simulink model "wetmodel"  (R2019b)
settings: Solver=ode45  StartTime=0.0  StopTime=10  RelTol=1e-3  EnableMultiTasking=on
model workspace (MAT data in the model file):
  SB_TRANSCOEFF = [1 10.1 101]
values from neighbouring files (symbols this model uses):
  B_thruster = [pi/2 0.05 0]    [Model_driver.m]
  Kd_x = 0    [Model_driver.m]
  Kd_y = 0    [Model_driver.m]
  Kd_yaw = 0    [Model_driver.m]
  Ki_x = 0    [Model_driver.m]
  Ki_y = 0    [Model_driver.m]
  Ki_yaw = 0    [Model_driver.m]
  Kp_x = 10    [Model_driver.m]
  Kp_y = 10    [Model_driver.m]
  Kp_yaw = 10    [Model_driver.m]
  P_thruster = [pi/2 -0.05 -0.05]    [Model_driver.m]
  SB_D = 10    [Model_driver.m]
  SB_I = 10    [Model_driver.m]
  SB_P = 10    [Model_driver.m]
  SB_thruster = [0 -0.05 0.05]    [Model_driver.m]
undefined symbols (not defined in the file or in its folder): IsPositionTracked, IsSkeletonTracked, JointDepthIndices, JointImageIndices, JointTrackingState, JointWorldCoordinates, magnitude, none, PositionDepthIndices, PositionImageIndices, PositionWorldCoordinates, Rec, SDTV, SegmentationData, SkeletonTrackingID, videoinput
libraries: powerlib_meascontrol x8, simulink x3, visionconversions x2, imaqlib x1, visionstatistics x1, visionsinks x1
settings Model: Tag=MP_system  Creator=Andries  LastModifiedBy=odend
settings DataIOCC: LimitDataPoints=on  SaveFormat=Array  SignalLoggingSaveFormat=ModelDataLogs  ReturnWorkspaceOutputs=off
settings OptimizationCC: ExpressionDepthLimit=2147483647  LifeSpan=inf
settings DebuggingCC: UnderspecifiedInitializationDetection=Classic  MergeDetectMultiDrivingBlocksExec=none  SolverPrmCheckMsg=warning  FcnCallInpInsideContextMsg=warning  StateNameClashWarn=warning  SFUnexpectedBacktrackingDiag=warning  SFNoUnconditionalDefaultTransitionDiag=warning  SFExecutionAtInitializationDiag=none  ArithmeticOperatorsInVariantConditions=warning
settings HardwareCC: ProdBitPerPointer=32  ProdBitPerSizeT=32  ProdBitPerPtrDiffT=32  ProdLargestAtomicFloat=None  ProdIntDivRoundTo=Undefined  ProdEndianess=Unspecified  ProdWordSize=32  ProdHWDeviceType=32-bit Generic
settings ModelReferenceCC: PropagateSignalLabelsOutOfModel=off
settings SFSimCC: SimUseLocalCustomCode=off  CustomCodeUndefinedFunction=UseInterfaceOnly
settings RTWCC: RTWUseLocalCustomCode=off
settings CodeAppCC: StateflowObjectComments=on
settings GRTTargetCC: TargetLangStandard=C89/C90 (ANSI)  GeneratePreprocessorConditionals=Disable all  CombineOutputUpdateFcns=off  GRTInterface=on
settings ConfigComp: CovMetricSettings=dw  CovHtmlReporting=on  CovSaveCumulativeToWorkspaceVar=on  CovSaveSingleToWorkspaceVar=on  CovExternalEMLEnable=off

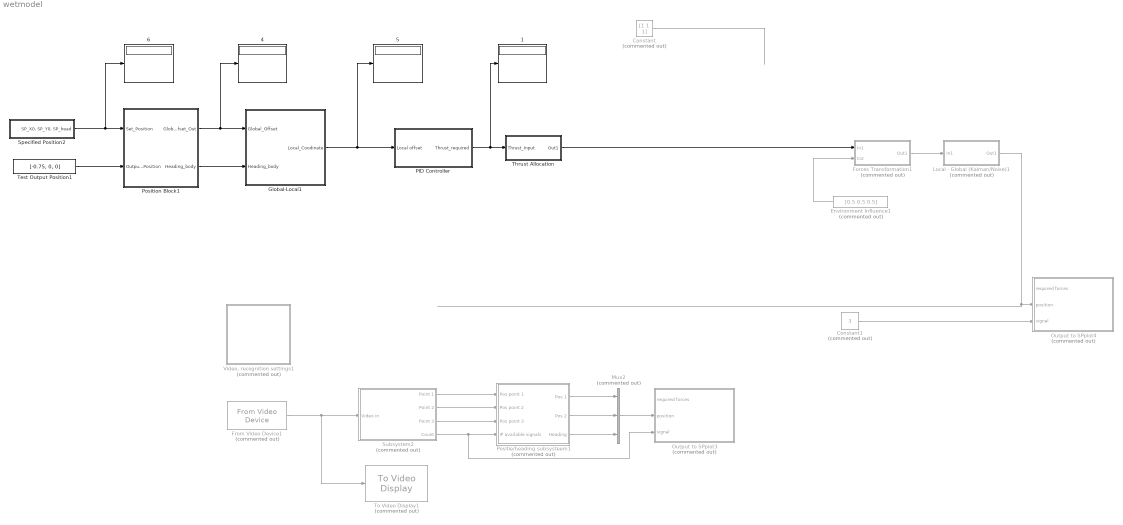
== system wetmodel ==
    {1,4..6} (4 alike) : Display
  Constant : Constant  Commented=on  Value=[1 1 1]
  Constant1 : Constant  Commented=on  Value=3
  Environment Influence1 : Constant  Commented=on  Value=[0.5 0.5 0.5]
  Forces Transformation1 : Subsystem  Commented=on
  From Video Device1 : imaqlib/From Video Device  Commented=on  DeviceMenu=(none)  Device=winvideo 1 (TOSHIBA Web Camera - HD)  ObjConstructor=videoinput('winvideo', 1)  VideoFormatMenu=(none)  VideoFormat=MJPG_1280x720  VideoSource=input1  ROIPosition=[0 0 720 1280]  EnableHWTrigger=off  TriggerConfiguration=none/none  SampleTime=1/30  OutputPortsMode=One multidimensional signal  DataType=single  CanDoHWTrigger=no  ReturnedColorSpace=rgb  BlockHandle=23.0015  ROIWidth=1280  ROIHeight=720  ROIColumn=0  ROIRow=0  EngXMLPath=C:\Program Files\MATLAB\R2019b\toolbox\imaq\imaq\private  DevXMLPath=C:\Program Files\MATLAB\R2013b\toolbox\imaq\imaqadaptors\win64  EngLibPath=C:\Program Files\MATLAB\R2019b\toolbox\imaq\imaqblks\imaqmex\win64  ColorSpace=rgb  BayerSensorAlignment=grbg  AllMetadata=IsPositionTracked;IsSkeletonTracked;JointDepthIndices;JointImageIndices;JointTrackingState;JointWorldCoordinates;PositionDepthIndices;PositionImageIndices;PositionWorldCoordinates;SegmentationData;SkeletonTrackingID  ImaqMode=off
      settings: SourceProductName=Image Acquisition Toolbox
  Global-Local1 : Subsystem
  Local - Global (Kalman/Noise)1 : Subsystem  Commented=on
  Mux2 : Mux  Commented=on  Inputs=3
  Output to SPplot3 : Subsystem  Commented=on
      mask Display:
      | image(imread('spplot.JPG'))
      | port_label('input', 1, 'Req. Forces')
      | port_label('input', 2, 'Pos Update')
      | port_label('input', 3, 'signal')
  Output to SPplot4 : Subsystem  Commented=on
      mask Display:
      | image(imread('spplot.JPG'))
      | port_label('input', 1, 'Req. Forces')
      | port_label('input', 2, 'Pos Update')
      | port_label('input', 3, 'signal')
  PID Controller : Subsystem
  Positie/heading subsysteem1 : Subsystem  Commented=on
  Position Block1 : Subsystem
  Specified Position2 : Subsystem
  Subsystem2 : Subsystem  Commented=on
  Test Output Position1 : Constant  Value=[-0.75, 0, 0]
  Thrust Allocation : Subsystem
  To Video Display1 : visionsinks/To Video Display  Commented=on  windowSizeMode=True size (1:1)  openAtMdlStart=on  fullScreen=off  videoWindowX=85  videoWindowY=2  saveWindowSize=off  videoWindowWidth=640  videoWindowHeight=480  inputColorFormat=RGB  inputType=Obsolete  imagePorts=One multidimensional signal  OutputDevice=On-screen video monitor  dataOrg=Column-major  isWindowOpen=on
      settings: SourceProductName=Computer Vision Toolbox
  "Video, recognition settings1" : Subsystem  Commented=on  mask{VG=1/290, X_off=-1, Y_off=.98, S_max=37, S_min=27}
      mask prompts: VG "Video Gain"; X_off "X offset"; Y_off "Y offset"; S_max "Signal Recognition Max"; S_min "Signal Recognition min"
      mask Display: text(.3, 0.5, 'Settings')
  wires:
  Forces Transformation1/1(Out1) -> Local - Global (Kalman/Noise)1/1(In1)
  Local - Global (Kalman/Noise)1/1(Out1) -> Output to SPplot4/2(position)
  Subsystem2/1(Point 1) -> Positie/heading subsysteem1/1(Pos point 1)
  Subsystem2/2(Point 2) -> Positie/heading subsysteem1/2(Pos point 2)
  Subsystem2/3(Point 3) -> Positie/heading subsysteem1/3(Pos point 3)
  Positie/heading subsysteem1/3(Heading) -> Mux2/3
  Positie/heading subsysteem1/1(Pos 1) -> Mux2/1
  Specified Position2/1("SP_X0, SP_Y0, SP_head") -> "  6"/1, Position Block1/1(Set_Position)
  Mux2/1 -> Output to SPplot3/2(position)
  From Video Device1/1 -> Subsystem2/1(Video in), To Video Display1/1
  Thrust Allocation/1(Out1) -> Forces Transformation1/1(In1)
  Environment Influence1/1 -> Forces Transformation1/2(In2)
  Test Output Position1/1 -> Position Block1/2(Output_Position)
  Positie/heading subsysteem1/2(Pos 2) -> Mux2/2
  Position Block1/1(Global_Offset_Out) -> "  4"/1, Global-Local1/1(Global_Offset)
  Subsystem2/4(Count) -> Output to SPplot3/3(signal), Positie/heading subsysteem1/4(# available signals)
  Global-Local1/1(Local_Coodinate) -> PID Controller/1(Local offset), "  5"/1
  Constant1/1 -> Output to SPplot4/3(signal)
  Position Block1/2(Heading_body) -> Global-Local1/2(Heading_body)
  Constant/1 -> ?
  PID Controller/1(Thrust_required) -> "  1"/1, Thrust Allocation/1(Thrust_Input)

== system wetmodel/Forces Transformation1 ==
  In1 : Inport
  In2 : Inport  Port=2
  Out1 : Outport

== system wetmodel/Global-Local1 ==
  Global_Offset : Inport
  Heading_body : Inport  Port=2
  Demux : Demux  Outputs=3
  Mux : Mux  Inputs=2
  Rotation Matrix : Subsystem
  Subsystem : Subsystem
  Local_Coodinate : Outport
  wires:
  Global_Offset/1 -> Demux/1
  Demux/1 -> Rotation Matrix/1(xinput)
  Demux/2 -> Rotation Matrix/2(yinput)
  Rotation Matrix/1(Rotation_Output) -> Mux/1
  Mux/1 -> Local_Coodinate/1
  Demux/3 -> Subsystem/1(Heading_Global_Offset)
  Subsystem/1("Heading_Local_Offset ") -> Mux/2
  Heading_body/1 -> Rotation Matrix/3(Heading_body)

== system wetmodel/Local - Global (Kalman//Noise)1 ==
  In1 : Inport
  Out1 : Outport
  wires:
  In1/1 -> Out1/1

== system wetmodel/Output to SPplot3 ==
  required forces : Inport
  position : Inport  Port=2
  signal : Inport  Port=3
  Constant : Constant  Value=3
  Mux : Mux  Inputs=3
  Switch : Switch  Criteria=u2 > Threshold
  pos_update : S-Function  FunctionName=pos_update  Parameters=TS_wii  SFunctionDeploymentMode=off  EnableBusSupport=off
  wires:
  Mux/1 -> pos_update/1
  position/1 -> Mux/1
  required forces/1 -> Mux/3
  Switch/1 -> Mux/2
  signal/1 -> Switch/2
  Constant/1 -> Switch/1

== system wetmodel/Output to SPplot4 ==
  required forces : Inport
  position : Inport  Port=2
  signal : Inport  Port=3
  Constant : Constant  Value=3
  Mux : Mux  Inputs=3
  Switch : Switch  Criteria=u2 > Threshold
  pos_update : S-Function  FunctionName=pos_update  Parameters=TS_wii  SFunctionDeploymentMode=off  EnableBusSupport=off
  wires:
  Mux/1 -> pos_update/1
  position/1 -> Mux/1
  required forces/1 -> Mux/3
  Switch/1 -> Mux/2
  signal/1 -> Switch/2
  Constant/1 -> Switch/1

== system wetmodel/PID Controller ==
  Local offset : Inport
  Demux : Demux  Outputs=3
  Mux : Mux  Inputs=3
  X Thrust PID : Subsystem
  X_output : Scope
  Y Thrust PID : Subsystem
  Y_output : Scope
  Yaw Angle PID : Subsystem
  Yaw_output : Scope
  Thrust_required : Outport
  wires:
  Local offset/1 -> Demux/1
  Demux/1 -> X Thrust PID/1(x_offset)
  Demux/2 -> Y Thrust PID/1(y_offset)
  Demux/3 -> Yaw Angle PID/1(yaw_offset)
  Mux/1 -> Thrust_required/1
  X Thrust PID/1(x_thrust_required) -> Mux/1, X_output/1
  Y Thrust PID/1(y_thrust_required) -> Mux/2, Y_output/1
  Yaw Angle PID/1(Yaw_moment_required) -> Mux/3, Yaw_output/1

== system wetmodel/Positie//heading subsysteem1 ==
  Pos point 1 : Inport
  Pos point 2 : Inport  Port=2
  Pos point 3 : Inport  Port=3
  # available signals : Inport  Port=4
  "Heading subsysteem " : Subsystem
  "Positie subsysteem . " : Subsystem
  Pos 1 : Outport
  Pos 2 : Outport  Port=2
  Heading : Outport  Port=3
  wires:
  Pos point 1/1 -> "Heading subsysteem "/1(In1), "Positie subsysteem . "/1(In1)
  Pos point 2/1 -> "Heading subsysteem "/2(In2), "Positie subsysteem . "/2(In2)
  "Positie subsysteem . "/2(pos 2) -> Pos 2/1
  "Positie subsysteem . "/1(pos 1) -> Pos 1/1
  Pos point 3/1 -> "Heading subsysteem "/3(In3), "Positie subsysteem . "/3(In3)
  # available signals/1 -> "Heading subsysteem "/4(In4), "Positie subsysteem . "/4(In4)
  "Heading subsysteem "/1(Heading) -> Heading/1

== system wetmodel/Position Block1 ==
  Set_Position : Inport
  Output_Position : Inport  Port=2
  Subtract : Sum  Inputs=+-
  Global_Offset_Out : Outport
  Heading_body : Outport  Port=2
  wires:
  Set_Position/1 -> Subtract/1
  Output_Position/1 -> Heading_body/1, Subtract/2
  Subtract/1 -> Global_Offset_Out/1

== system wetmodel/Specified Position2 ==
  Mux : Mux  Inputs=3
  SP_X0 : Constant  Value=0
  SP_Y0 : Constant  Value=0
  SP_head : Constant  Value=0
  "SP_X0, SP_Y0, SP_head" : Outport
  wires:
  Mux/1 -> "SP_X0, SP_Y0, SP_head"/1
  SP_Y0/1 -> Mux/2  "SP_Y0"
  SP_X0/1 -> Mux/1  "SP_X0"
  SP_head/1 -> Mux/3

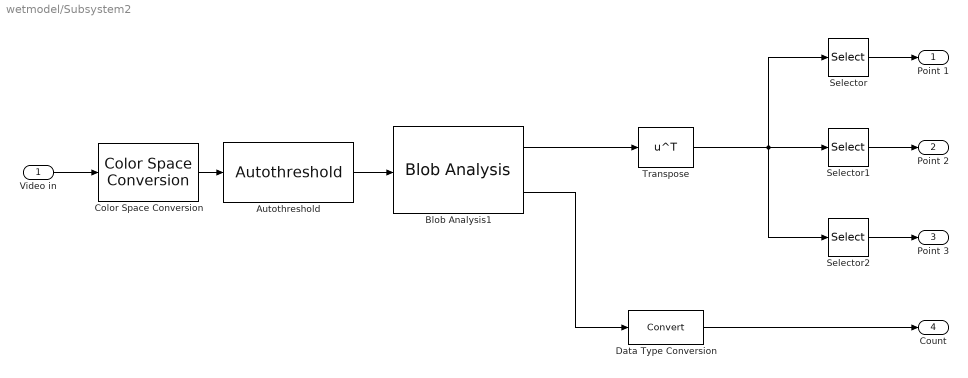
== system wetmodel/Subsystem2 ==
  Video in : Inport
  Autothreshold : visionconversions/Autothreshold  operator=>  threshOut=off  effMetricOut=off  userDefinedRange=on  umin=0.07  umax=1  outOfRngOpt=Ignore  scaleThreshold=off  scaleFactor=1  roundingMode=Floor  overflowMode=off  P1Mode=Slope and bias scaling  P1WordLength=32  P1FracLength=30  P1Slope=2^-30  A1Slope=2^-30  P2Mode=Specify word length  P2WordLength=32  P2FracLength=22  P2Slope=2^-22  A2Slope=2^-22  P3Mode=Specify word length  P3WordLength=32  P3FracLength=14  P3Slope=2^-14  A3Slope=2^-14  P4Mode=Binary point scaling  P4WordLength=32  P4FracLength=15  P4Slope=2^-15  A4Slope=2^-4  Q1Mode=Specify word length  Q1WordLength=32  Q1FracLength=16  Q1Slope=2^-16  EMMode=Specify word length  EMWordLength=16  EMFracLength=14  EMSlope=2^-14
      settings: SourceProductName=Computer Vision Toolbox  SourceProductBaseCode=VP
  Blob Analysis1 : visionstatistics/Blob Analysis  Tag=vipblks_row_conv  area=off  centroid=on  bBox=off  majorAxis=off  minorAxis=off  angle=off  eccentricity=off  equivDiameterSq=off  extent=off  perimeter=off  outDT=single  conn=8  isLabel=off  maxBlobs=3  warnIfNumBlobsExceeded=off  isCount=on  useMinArea=on  minArea=20  useMaxArea=on  maxArea=300  excludeBorderBlob=off  isOutVarDim=off  isFill=on  fillValues=-1  roundingMode=Floor  overflowMode=off  prodOutputMode=Binary point scaling  prodOutputWordLength=32  prodOutputFracLength=16  prodOutputSlope=2^-16  accumMode=Binary point scaling  accumWordLength=32  accumFracLength=0  accumSlope=2^0  outputMode=Binary point scaling  outputWordLength=32  outputFracLength=16  outputSlope=2^-16  memorySlope=2^-16  firstCoeffMode=Binary point scaling  firstCoeffWordLength=16  firstCoeffFracLength=14  firstCoeffSlope=2^-14  secondCoeffMode=Binary point scaling  secondCoeffWordLength=32  secondCoeffFracLength=16  secondCoeffSlope=2^-16
      settings: SourceProductName=Computer Vision Toolbox
  Color Space Conversion : visionconversions/Color Space  Conversion  conversion=Obsolete  conversionActive=R'G'B' to intensity  wp_str=D65  rec=Rec. 601 (SDTV)  sys=1125/60/2:1  imagePorts=One multidimensional signal
  Data Type Conversion : DataTypeConversion
  Selector : Selector  NumberOfDimensions=2  InputPortWidth=3  IndexOptions=Select all,Index vector (dialog)  Indices=[1 3],1  OutputSizes=1,1
  Selector1 : Selector  NumberOfDimensions=2  InputPortWidth=3  IndexOptions=Select all,Index vector (dialog)  Indices=[1 3],2  OutputSizes=1,1
  Selector2 : Selector  NumberOfDimensions=2  InputPortWidth=3  IndexOptions=Select all,Index vector (dialog)  Indices=[1 3],3  OutputSizes=1,1
  Transpose : Math  Operator=transpose  SignedPower=off  SaturateOnIntegerOverflow=on
  Point 1 : Outport
  Point 2 : Outport  Port=2
  Point 3 : Outport  Port=3
  Count : Outport  Port=4
  wires:
  Autothreshold/1 -> Blob Analysis1/1
  Color Space Conversion/1 -> Autothreshold/1
  Video in/1 -> Color Space Conversion/1
  Blob Analysis1/2 -> Data Type Conversion/1
  Selector/1 -> Point 1/1
  Selector1/1 -> Point 2/1
  Selector2/1 -> Point 3/1
  Blob Analysis1/1 -> Transpose/1
  Transpose/1 -> Selector/1, Selector2/1, Selector1/1
  Data Type Conversion/1 -> Count/1

== system wetmodel/Thrust Allocation ==
  Thrust_Input : Inport
  "  1" : Display
  Add : Sum  Inputs=+++
  Azimuth Thrust Allocation (Port) : Subsystem
  Azimuth Thrust Allocation (Starboard) : Subsystem
  Bow Thrust Allocation (Bow) : Subsystem
  DCMOTOR_Starboard : Subsystem
  Out1 : Outport
  wires:
  Thrust_Input/1 -> Bow Thrust Allocation (Bow)/1(Thrust_Input), Azimuth Thrust Allocation (Port)/1(Thrust_Input), Azimuth Thrust Allocation (Starboard)/1(Thrust_Input)
  Bow Thrust Allocation (Bow)/1(Bow_Output) -> Add/3
  Azimuth Thrust Allocation (Port)/1(Azimuth_P_Output) -> Add/2
  Azimuth Thrust Allocation (Starboard)/1(Azimuth_SB_Output) -> Add/1
  Add/1 -> Out1/1, "  1"/1

== system wetmodel/Video, recognition settings1 ==
  "Signal recognition max " : Constant  Value=S_max
  Signal recognition min : Constant  Value=S_min
  Video gain : Constant  Value=VG
  "X offset " : Constant  Value=X_off
  "Y offset " : Constant  Value=Y_off
  tag scope: A=global, B=global, C=global, D=global, F=global
  wires:
  "X offset "/1 -> [A]
  Video gain/1 -> [C]
  "Y offset "/1 -> [B]
  Signal recognition min/1 -> [F]
  "Signal recognition max "/1 -> [D]

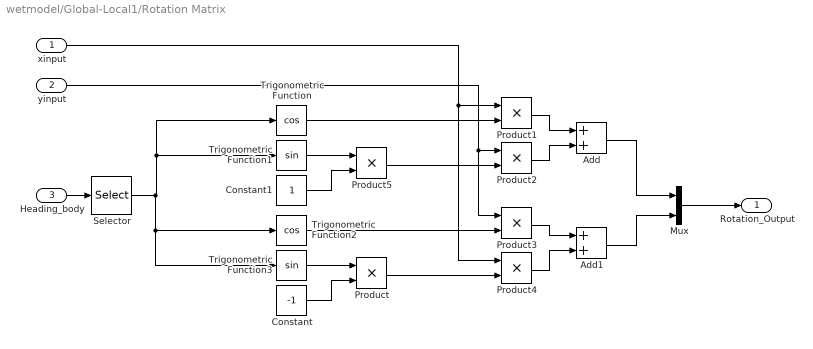
== system wetmodel/Global-Local1/Rotation Matrix ==
  xinput : Inport
  yinput : Inport  Port=2
  Heading_body : Inport  Port=3
  Add : Sum
  Add1 : Sum
  Constant : Constant  Value=-1
  Constant1 : Constant
  Mux : Mux  Inputs=2
  Product{,1..5} (6 alike) : Product
  Selector : Selector  InputPortWidth=3  IndexOptions=Starting index (dialog)  Indices=[ 3]  OutputSizes=1
  Trigonometric Function : Trigonometry  Operator=cos
  Trigonometric Function1 : Trigonometry
  Trigonometric Function2 : Trigonometry  Operator=cos
  Trigonometric Function3 : Trigonometry
  Rotation_Output : Outport
  wires:
  Selector/1 -> Trigonometric Function2/1, Trigonometric Function3/1, Trigonometric Function/1, Trigonometric Function1/1
  Trigonometric Function3/1 -> Product/1
  Trigonometric Function1/1 -> Product5/1
  Trigonometric Function/1 -> Product1/2
  Constant/1 -> Product/2
  xinput/1 -> Product4/1, Product1/1
  yinput/1 -> Product3/1, Product2/1
  Product/1 -> Product4/2
  Trigonometric Function2/1 -> Product3/2
  Product1/1 -> Add/1
  Product2/1 -> Add/2
  Add/1 -> Mux/1
  Add1/1 -> Mux/2
  Product4/1 -> Add1/2
  Product3/1 -> Add1/1
  Mux/1 -> Rotation_Output/1
  Constant1/1 -> Product5/2
  Product5/1 -> Product2/2
  Heading_body/1 -> Selector/1

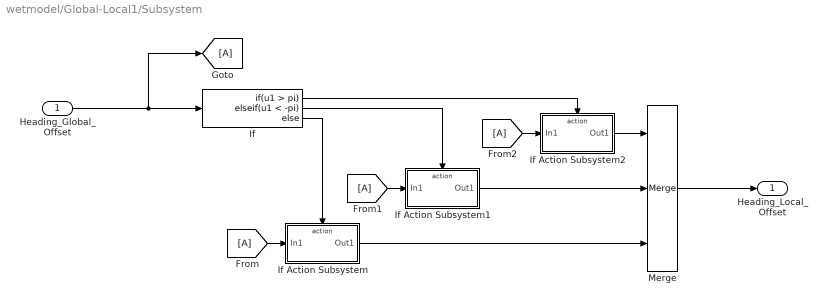
== system wetmodel/Global-Local1/Subsystem ==
  Heading_Global_Offset : Inport
  If : If  IfExpression=u1 > pi  ElseIfExpressions=u1 < -pi
  If Action Subsystem : Subsystem  TreatAsAtomicUnit=on
  If Action Subsystem1 : Subsystem  TreatAsAtomicUnit=on
  If Action Subsystem2 : Subsystem  TreatAsAtomicUnit=on
  Merge : Merge  Inputs=3
  "Heading_Local_Offset " : Outport
  wires:
  Heading_Global_Offset/1 -> If/1, [A]
  If Action Subsystem1/1(Out1) -> Merge/2
  [A] -> If Action Subsystem/1(In1)
  If Action Subsystem2/1(Out1) -> Merge/1
  [A] -> If Action Subsystem2/1(In1)
  [A] -> If Action Subsystem1/1(In1)
  If/1 -> If Action Subsystem2/Action
  If/3 -> If Action Subsystem/Action
  If/2 -> If Action Subsystem1/Action
  If Action Subsystem/1(Out1) -> Merge/3
  Merge/1 -> "Heading_Local_Offset "/1

== system wetmodel/PID Controller/X Thrust PID ==
  x_offset : Inport
  Add : Sum  Inputs=+++
  Derivative : Derivative
  Gain : Gain  Gain=Ki_x
  Gain1 : Gain  Gain=Kd_x
  Gain2 : Gain  Gain=Kp_x
  Integrator : Integrator
  Saturation : Saturate  UpperLimit=1  LowerLimit=-1
  x_thrust_required : Outport
  wires:
  Add/1 -> Saturation/1
  Derivative/1 -> Gain1/1
  x_offset/1 -> Gain2/1, Derivative/1, Integrator/1
  Integrator/1 -> Gain/1
  Gain/1 -> Add/1
  Gain1/1 -> Add/2
  Gain2/1 -> Add/3
  Saturation/1 -> x_thrust_required/1

== system wetmodel/PID Controller/Y Thrust PID ==
  y_offset : Inport
  Add : Sum  Inputs=+++
  Derivative : Derivative
  Gain : Gain  Gain=Ki_y
  Gain1 : Gain  Gain=Kd_y
  Gain2 : Gain  Gain=Kp_y
  Integrator : Integrator
  Saturation : Saturate  UpperLimit=1  LowerLimit=-1
  y_thrust_required : Outport
  wires:
  Add/1 -> Saturation/1
  Derivative/1 -> Gain1/1
  y_offset/1 -> Gain2/1, Derivative/1, Integrator/1
  Integrator/1 -> Gain/1
  Gain/1 -> Add/1
  Gain1/1 -> Add/2
  Gain2/1 -> Add/3
  Saturation/1 -> y_thrust_required/1

== system wetmodel/PID Controller/Yaw Angle PID ==
  yaw_offset : Inport
  Add : Sum  Inputs=+++
  Derivative : Derivative
  Gain : Gain  Gain=Ki_yaw
  Gain1 : Gain  Gain=Kp_yaw
  Gain3 : Gain  Gain=Kd_yaw
  Integrator : Integrator
  Saturation : Saturate  UpperLimit=1  LowerLimit=-1
  Yaw_moment_required : Outport
  wires:
  Add/1 -> Saturation/1
  yaw_offset/1 -> Gain1/1, Derivative/1, Integrator/1
  Integrator/1 -> Gain/1
  Gain/1 -> Add/1
  Derivative/1 -> Gain3/1
  Gain3/1 -> Add/2
  Gain1/1 -> Add/3
  Saturation/1 -> Yaw_moment_required/1

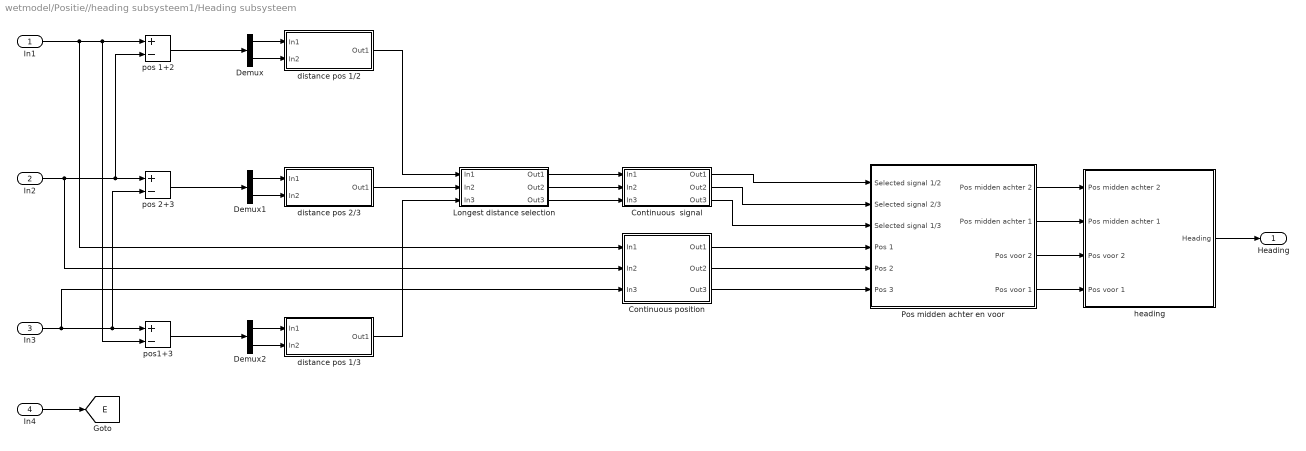
== system wetmodel/Positie//heading subsysteem1/Heading subsysteem  ==
  In1 : Inport
  In2 : Inport  Port=2
  In3 : Inport  Port=3
  In4 : Inport  Port=4
  Continuous position : Subsystem
  Continuous  signal : Subsystem
  Demux : Demux  Outputs=2
  Demux1 : Demux  Outputs=2
  Demux2 : Demux  Outputs=2
  "Longest distance selection " : Subsystem
  "Pos midden achter en voor " : Subsystem
  "distance pos 1/2 " : Subsystem
  "distance pos 1/3 " : Subsystem
  "distance pos 2/3 " : Subsystem
  heading : Subsystem
  "pos 1+2 " : Sum  Inputs=+-
  "pos 2+3 " : Sum  Inputs=+-
  "pos1+3 " : Sum  Inputs=+-
  Heading : Outport
  tag scope: E=global
  wires:
  "pos 1+2 "/1 -> Demux/1
  "pos 2+3 "/1 -> Demux1/1
  "pos1+3 "/1 -> Demux2/1
  Demux/1 -> "distance pos 1/2 "/1(In1)
  Demux/2 -> "distance pos 1/2 "/2(In2)
  Demux1/1 -> "distance pos 2/3 "/1(In1)
  Demux1/2 -> "distance pos 2/3 "/2(In2)
  Demux2/2 -> "distance pos 1/3 "/2(In2)
  Demux2/1 -> "distance pos 1/3 "/1(In1)
  "distance pos 1/2 "/1(Out1) -> "Longest distance selection "/1(In1)
  "distance pos 1/3 "/1(Out1) -> "Longest distance selection "/3(In3)
  "distance pos 2/3 "/1(Out1) -> "Longest distance selection "/2(In2)
  "Longest distance selection "/2(Out2) -> Continuous  signal/2(In2)
  "Longest distance selection "/3(Out3) -> Continuous  signal/3(In3)
  "Longest distance selection "/1(Out1) -> Continuous  signal/1(In1)
  In1/1 -> Continuous position/1(In1), "pos1+3 "/2, "pos 1+2 "/1
  In2/1 -> Continuous position/2(In2), "pos 2+3 "/1, "pos 1+2 "/2
  In3/1 -> Continuous position/3(In3), "pos1+3 "/1, "pos 2+3 "/2
  Continuous  signal/1(Out1) -> "Pos midden achter en voor "/1("Selected signal 1/2 ")
  Continuous  signal/2(Out2) -> "Pos midden achter en voor "/2("Selected signal 2/3 ")
  Continuous  signal/3(Out3) -> "Pos midden achter en voor "/3(Selected signal 1/3)
  Continuous position/1(Out1) -> "Pos midden achter en voor "/4("Pos 1 ")
  Continuous position/2(Out2) -> "Pos midden achter en voor "/5(Pos 2)
  Continuous position/3(Out3) -> "Pos midden achter en voor "/6(Pos 3)
  "Pos midden achter en voor "/1(Pos midden achter 2) -> heading/1(Pos midden achter 2)
  "Pos midden achter en voor "/2(Pos midden achter 1) -> heading/2(Pos midden achter 1)
  "Pos midden achter en voor "/3("Pos voor 2 ") -> heading/3("Pos voor 2 ")
  "Pos midden achter en voor "/4(Pos voor 1) -> heading/4(Pos voor 1)
  heading/1(Heading) -> Heading/1
  In4/1 -> [E]

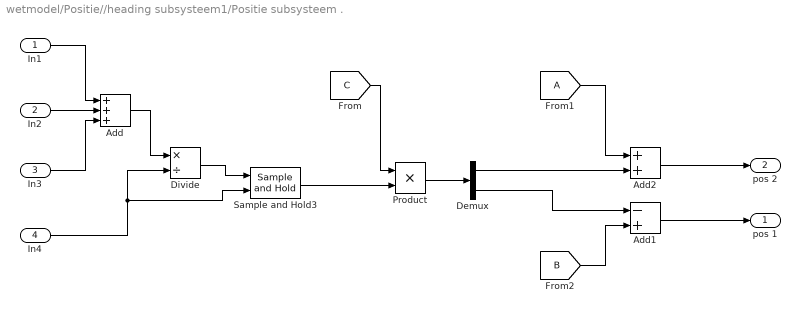
== system wetmodel/Positie//heading subsysteem1/Positie subsysteem .  ==
  In1 : Inport
  In2 : Inport  Port=2
  In3 : Inport  Port=3
  In4 : Inport  Port=4
  Add : Sum  Inputs=+++
  Add1 : Sum  Inputs=-+
  Add2 : Sum
  Demux : Demux  Outputs=2
  Divide : Product  Inputs=*/
  Product : Product
  Sample and Hold3 : powerlib_meascontrol/Additional Components/Sample and Hold  ic=0  Ts=0
      settings: SourceProductName=Simscape Electrical  SourceProductBaseCode=PS
  pos 1 : Outport
  pos 2 : Outport  Port=2
  wires:
  Divide/1 -> Sample and Hold3/1
  In1/1 -> Add/1
  In2/1 -> Add/2
  In3/1 -> Add/3
  Add/1 -> Divide/1
  In4/1 -> Sample and Hold3/2, Divide/2
  Add1/1 -> pos 1/1
  Sample and Hold3/1 -> Product/2
  Product/1 -> Demux/1
  Demux/1 -> Add2/2
  Demux/2 -> Add1/1
  Add2/1 -> pos 2/1
  [C] -> Product/1
  [A] -> Add2/1
  [B] -> Add1/2

== system wetmodel/Thrust Allocation/Azimuth Thrust Allocation (Port) ==
  Thrust_Input : Inport
  " " : Constant  Value=P_thruster
  Display : Display
  Moment : Fcn  Expr=-u(3)*cos(u(1))+u(2)*sin(u(1))
  Mux : Mux  Inputs=3
  Product : Product
  Selector : Selector  InputPortWidth=3  IndexOptions=Index vector (dialog)  Indices=[1]  OutputSizes=1
  Trigonometric Function : Trigonometry  Operator=cos
  Trigonometric Function1 : Trigonometry
  Azimuth_P_Output : Outport
  wires:
  Moment/1 -> Mux/3
  Trigonometric Function/1 -> Mux/1
  " "/1 -> Moment/1, Selector/1
  Selector/1 -> Trigonometric Function/1, Trigonometric Function1/1
  Trigonometric Function1/1 -> Mux/2
  Thrust_Input/1 -> Product/2
  Mux/1 -> Product/1
  Product/1 -> Display/1, Azimuth_P_Output/1

== system wetmodel/Thrust Allocation/Azimuth Thrust Allocation (Starboard) ==
  Thrust_Input : Inport
  " " : Constant  Value=SB_thruster
  Display : Display
      settings: Format=short_e
  Moment : Fcn  Expr=-u(3)*cos(u(1))+u(2)*sin(u(1))
  Mux : Mux  Inputs=3
  Product : Product
  Selector : Selector  InputPortWidth=3  IndexOptions=Index vector (dialog)  Indices=[1]  OutputSizes=1
  Trigonometric Function : Trigonometry  Operator=cos
  Trigonometric Function1 : Trigonometry
  Azimuth_SB_Output : Outport
  wires:
  Moment/1 -> Mux/3
  Trigonometric Function/1 -> Mux/1
  " "/1 -> Moment/1, Selector/1
  Selector/1 -> Trigonometric Function/1, Trigonometric Function1/1
  Trigonometric Function1/1 -> Mux/2
  Thrust_Input/1 -> Product/2
  Mux/1 -> Product/1
  Product/1 -> Display/1, Azimuth_SB_Output/1

== system wetmodel/Thrust Allocation/Bow Thrust Allocation (Bow) ==
  Thrust_Input : Inport
  " " : Constant  Value=B_thruster
  Display : Display
  Moment : Fcn  Expr=-u(3)*cos(u(1))+u(2)*sin(u(1))
  Mux : Mux  Inputs=3
  Product : Product
  Selector : Selector  InputPortWidth=3  IndexOptions=Index vector (dialog)  Indices=[1]  OutputSizes=1
  Trigonometric Function : Trigonometry  Operator=cos
  Trigonometric Function1 : Trigonometry
  Bow_Output : Outport
  wires:
  Moment/1 -> Mux/3
  Trigonometric Function/1 -> Mux/1
  " "/1 -> Moment/1, Selector/1
  Selector/1 -> Trigonometric Function/1, Trigonometric Function1/1
  Trigonometric Function1/1 -> Mux/2
  Thrust_Input/1 -> Product/2
  Mux/1 -> Product/1
  Product/1 -> Display/1, Bow_Output/1

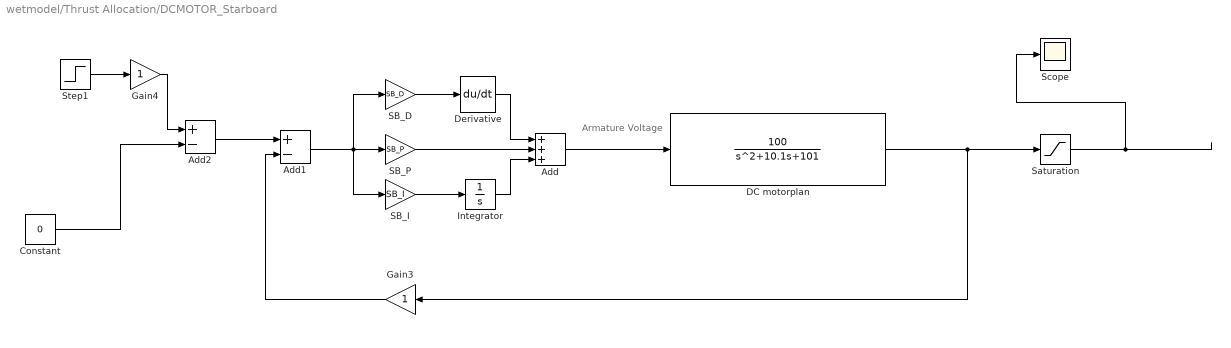
== system wetmodel/Thrust Allocation/DCMOTOR_Starboard ==
  note: Armature Voltage
  Add : Sum  Inputs=+++
  Add1 : Sum  Inputs=+-
  Add2 : Sum  Inputs=+-
  Constant : Constant  Value=0
  DC motorplan : TransferFcn  Numerator=100  Denominator=[1 10.1 101]
  Derivative : Derivative
  Gain3 : Gain
  Gain4 : Gain
  Integrator : Integrator
  SB_D : Gain  Gain=SB_D
  SB_I : Gain  Gain=SB_I
  SB_P : Gain  Gain=SB_P
  Saturation : Saturate
  Scope : Scope
  Step1 : Step  Time=2  SampleTime=0
  wires:
  SB_I/1 -> Integrator/1
  SB_P/1 -> Add/2
  Add/1 -> DC motorplan/1
  Derivative/1 -> Add/1
  Integrator/1 -> Add/3
  Add1/1 -> SB_I/1, SB_D/1, SB_P/1
  SB_D/1 -> Derivative/1
  Gain3/1 -> Add1/2
  Add2/1 -> Add1/1
  Step1/1 -> Gain4/1
  Gain4/1 -> Add2/1
  Constant/1 -> Add2/2
  DC motorplan/1 -> Gain3/1, Saturation/1
  Saturation/1 -> Scope/1

== system wetmodel/Global-Local1/Subsystem/If Action Subsystem ==
  In1 : Inport
  Action Port : ActionPort  ActionPortLabel=else
  Out1 : Outport
  wires:
  In1/1 -> Out1/1

== system wetmodel/Global-Local1/Subsystem/If Action Subsystem1 ==
  In1 : Inport
  Action Port : ActionPort  ActionPortLabel=elseif(u1 < -pi)
  Add : Sum
  Constant : Constant  Value=2*pi
  Out1 : Outport
  wires:
  In1/1 -> Add/1
  Constant/1 -> Add/2
  Add/1 -> Out1/1

== system wetmodel/Global-Local1/Subsystem/If Action Subsystem2 ==
  In1 : Inport
  Action Port : ActionPort  ActionPortLabel=if(u1 > pi)
  Constant : Constant  Value=2*pi
  Subtract : Sum  Inputs=+-
  Out1 : Outport
  wires:
  In1/1 -> Subtract/1
  Constant/1 -> Subtract/2
  Subtract/1 -> Out1/1

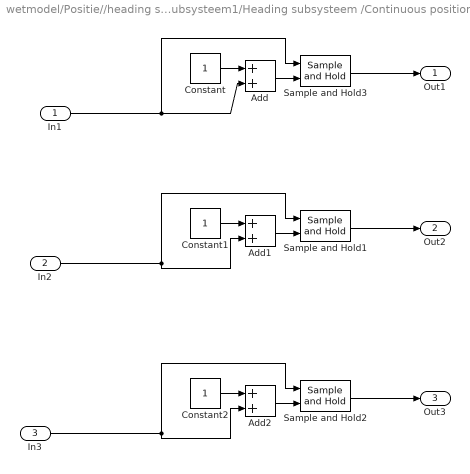
== system wetmodel/Positie//heading subsysteem1/Heading subsysteem /Continuous position ==
  In1 : Inport
  In2 : Inport  Port=2
  In3 : Inport  Port=3
  Add : Sum
  Add1 : Sum
  Add2 : Sum
  Constant : Constant
  Constant1 : Constant
  Constant2 : Constant
  Sample and Hold1 : powerlib_meascontrol/Additional Components/Sample and Hold  ic=0  Ts=0
      settings: SourceProductName=Simscape Electrical  SourceProductBaseCode=PS
  Sample and Hold2 : powerlib_meascontrol/Additional Components/Sample and Hold  ic=0  Ts=0
      settings: SourceProductName=Simscape Electrical  SourceProductBaseCode=PS
  Sample and Hold3 : powerlib_meascontrol/Additional Components/Sample and Hold  ic=0  Ts=0
      settings: SourceProductName=Simscape Electrical  SourceProductBaseCode=PS
  Out1 : Outport
  Out2 : Outport  Port=2
  Out3 : Outport  Port=3
  wires:
  Add/1 -> Sample and Hold3/2
  Constant/1 -> Add/1
  In1/1 -> Sample and Hold3/1, Add/2
  Add1/1 -> Sample and Hold1/2
  Constant1/1 -> Add1/1
  In2/1 -> Add1/2, Sample and Hold1/1
  Add2/1 -> Sample and Hold2/2
  Constant2/1 -> Add2/1
  In3/1 -> Add2/2, Sample and Hold2/1
  Sample and Hold3/1 -> Out1/1
  Sample and Hold2/1 -> Out3/1
  Sample and Hold1/1 -> Out2/1

== system wetmodel/Positie//heading subsysteem1/Heading subsysteem /Continuous  signal ==
  In1 : Inport
  In2 : Inport  Port=2
  In3 : Inport  Port=3
  Add1 : Sum  Inputs=+++
  Sample and Hold : powerlib_meascontrol/Additional Components/Sample and Hold  ic=0  Ts=0
      settings: SourceProductName=Simscape Electrical  SourceProductBaseCode=PS
  Sample and Hold1 : powerlib_meascontrol/Additional Components/Sample and Hold  ic=0  Ts=0
      settings: SourceProductName=Simscape Electrical  SourceProductBaseCode=PS
  Sample and Hold2 : powerlib_meascontrol/Additional Components/Sample and Hold  ic=0  Ts=0
      settings: SourceProductName=Simscape Electrical  SourceProductBaseCode=PS
  Out1 : Outport
  Out2 : Outport  Port=2
  Out3 : Outport  Port=3
  wires:
  In1/1 -> Add1/1, Sample and Hold/1
  Sample and Hold/1 -> Out1/1
  In2/1 -> Sample and Hold1/1, Add1/2
  In3/1 -> Sample and Hold2/1, Add1/3
  Add1/1 -> Sample and Hold2/2, Sample and Hold1/2, Sample and Hold/2
  Sample and Hold2/1 -> Out3/1
  Sample and Hold1/1 -> Out2/1

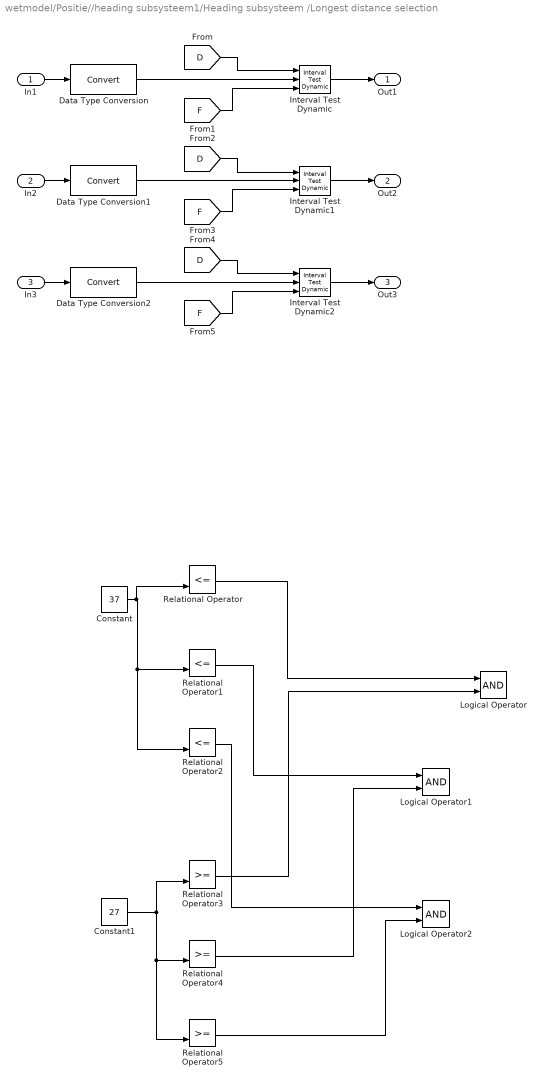
== system wetmodel/Positie//heading subsysteem1/Heading subsysteem /Longest distance selection  ==
  In1 : Inport
  In2 : Inport  Port=2
  In3 : Inport  Port=3
  Constant : Constant  Value=37
  Constant1 : Constant  Value=27
  Data Type Conversion : DataTypeConversion
  Data Type Conversion1 : DataTypeConversion
  Data Type Conversion2 : DataTypeConversion
  Interval Test Dynamic : simulink/Logic and Bit Operations/Interval Test Dynamic  IntervalClosedRight=on  IntervalClosedLeft=on  OutDataTypeStr=boolean
      settings: SourceProductName=Simulink  SourceProductBaseCode=SL
  Interval Test Dynamic1 : simulink/Logic and Bit Operations/Interval Test Dynamic  IntervalClosedRight=on  IntervalClosedLeft=on  OutDataTypeStr=boolean
      settings: SourceProductName=Simulink  SourceProductBaseCode=SL
  Interval Test Dynamic2 : simulink/Logic and Bit Operations/Interval Test Dynamic  IntervalClosedRight=on  IntervalClosedLeft=on  OutDataTypeStr=boolean
      settings: SourceProductName=Simulink  SourceProductBaseCode=SL
  Logical Operator : Logic  AllPortsSameDT=off  OutDataTypeStr=boolean
  Logical Operator1 : Logic  AllPortsSameDT=off  OutDataTypeStr=boolean
  Logical Operator2 : Logic  AllPortsSameDT=off  OutDataTypeStr=boolean
  Relational Operator : RelationalOperator  Operator=<=  OutDataTypeStr=boolean  RndMeth=Nearest
  Relational Operator1 : RelationalOperator  Operator=<=  OutDataTypeStr=boolean  RndMeth=Nearest
  Relational Operator2 : RelationalOperator  Operator=<=  OutDataTypeStr=boolean  RndMeth=Nearest
  Relational Operator3 : RelationalOperator  OutDataTypeStr=boolean  RndMeth=Nearest
  Relational Operator4 : RelationalOperator  OutDataTypeStr=boolean  RndMeth=Nearest
  Relational Operator5 : RelationalOperator  OutDataTypeStr=boolean  RndMeth=Nearest
  Out1 : Outport
  Out2 : Outport  Port=2
  Out3 : Outport  Port=3
  wires:
  Constant/1 -> Relational Operator2/2, Relational Operator1/2, Relational Operator/2
  Constant1/1 -> Relational Operator4/2, Relational Operator5/2, Relational Operator3/2
  Relational Operator/1 -> Logical Operator/1
  Relational Operator1/1 -> Logical Operator1/1
  Relational Operator4/1 -> Logical Operator1/2
  Relational Operator2/1 -> Logical Operator2/1
  Relational Operator5/1 -> Logical Operator2/2
  Relational Operator3/1 -> Logical Operator/2
  In1/1 -> Data Type Conversion/1
  Interval Test Dynamic/1 -> Out1/1
  Interval Test Dynamic2/1 -> Out3/1
  Interval Test Dynamic1/1 -> Out2/1
  [D] -> Interval Test Dynamic/1
  [F] -> Interval Test Dynamic/3
  In2/1 -> Data Type Conversion1/1
  [D] -> Interval Test Dynamic1/1
  [F] -> Interval Test Dynamic1/3
  [D] -> Interval Test Dynamic2/1
  [F] -> Interval Test Dynamic2/3
  In3/1 -> Data Type Conversion2/1
  Data Type Conversion/1 -> Interval Test Dynamic/2
  Data Type Conversion1/1 -> Interval Test Dynamic1/2
  Data Type Conversion2/1 -> Interval Test Dynamic2/2

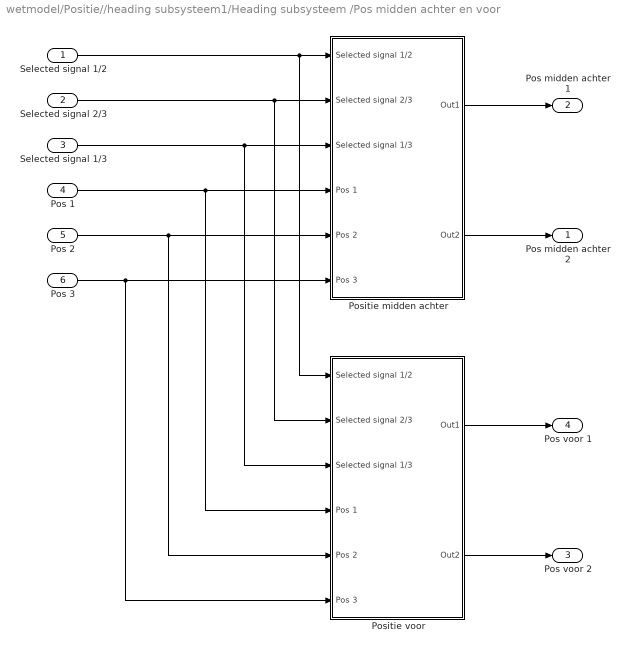
== system wetmodel/Positie//heading subsysteem1/Heading subsysteem /Pos midden achter en voor  ==
  "Selected signal 1/2 " : Inport
  "Selected signal 2/3 " : Inport  Port=2
  Selected signal 1/3 : Inport  Port=3
  "Pos 1 " : Inport  Port=4
  Pos 2 : Inport  Port=5
  Pos 3 : Inport  Port=6
  Positie midden achter : Subsystem
  Positie voor : Subsystem
  Pos midden achter 2 : Outport
  Pos midden achter 1 : Outport  Port=2
  "Pos voor 2 " : Outport  Port=3
  Pos voor 1 : Outport  Port=4
  wires:
  "Pos 1 "/1 -> Positie voor/4("Pos 1 "), Positie midden achter/4("Pos 1 ")
  Pos 2/1 -> Positie voor/5("Pos 2 "), Positie midden achter/5("Pos 2 ")
  Pos 3/1 -> Positie voor/6("Pos 3 "), Positie midden achter/6("Pos 3 ")
  Positie midden achter/1(Out1) -> Pos midden achter 1/1
  Positie midden achter/2(Out2) -> Pos midden achter 2/1
  "Selected signal 1/2 "/1 -> Positie voor/1(Selected signal 1/2), Positie midden achter/1(Selected signal 1/2)
  "Selected signal 2/3 "/1 -> Positie voor/2(Selected signal 2/3), Positie midden achter/2(Selected signal 2/3)
  Selected signal 1/3/1 -> Positie voor/3(Selected signal 1/3), Positie midden achter/3(Selected signal 1/3)
  Positie voor/1(Out1) -> Pos voor 1/1
  Positie voor/2(Out2) -> "Pos voor 2 "/1

== system wetmodel/Positie//heading subsysteem1/Heading subsysteem /distance pos 1//2  ==
  In1 : Inport
  In2 : Inport  Port=2
  Add : Sum
  Math Function : Math  Operator=magnitude^2  OutputSignalType=real  SaturateOnIntegerOverflow=on
  Math Function1 : Math  Operator=magnitude^2  OutputSignalType=real  SaturateOnIntegerOverflow=on
  Sqrt : Sqrt  SaturateOnIntegerOverflow=on
  Out1 : Outport
  wires:
  In1/1 -> Math Function/1
  In2/1 -> Math Function1/1
  Math Function/1 -> Add/1
  Math Function1/1 -> Add/2
  Add/1 -> Sqrt/1
  Sqrt/1 -> Out1/1

== system wetmodel/Positie//heading subsysteem1/Heading subsysteem /distance pos 1//3  ==
  In1 : Inport
  In2 : Inport  Port=2
  Add : Sum
  Math Function : Math  Operator=magnitude^2  OutputSignalType=real  SaturateOnIntegerOverflow=on
  Math Function1 : Math  Operator=magnitude^2  OutputSignalType=real  SaturateOnIntegerOverflow=on
  Sqrt : Sqrt  SaturateOnIntegerOverflow=on
  Out1 : Outport
  wires:
  In1/1 -> Math Function/1
  In2/1 -> Math Function1/1
  Math Function/1 -> Add/1
  Math Function1/1 -> Add/2
  Add/1 -> Sqrt/1
  Sqrt/1 -> Out1/1

== system wetmodel/Positie//heading subsysteem1/Heading subsysteem /distance pos 2//3  ==
  In1 : Inport
  In2 : Inport  Port=2
  Add : Sum
  Math Function : Math  Operator=magnitude^2  OutputSignalType=real  SaturateOnIntegerOverflow=on
  Math Function1 : Math  Operator=magnitude^2  OutputSignalType=real  SaturateOnIntegerOverflow=on
  Sqrt : Sqrt  SaturateOnIntegerOverflow=on
  Out1 : Outport
  wires:
  In1/1 -> Math Function/1
  In2/1 -> Math Function1/1
  Math Function/1 -> Add/1
  Math Function1/1 -> Add/2
  Add/1 -> Sqrt/1
  Sqrt/1 -> Out1/1

== system wetmodel/Positie//heading subsysteem1/Heading subsysteem /heading ==
  Pos midden achter 2 : Inport
  Pos midden achter 1 : Inport  Port=2
  "Pos voor 2 " : Inport  Port=3
  Pos voor 1 : Inport  Port=4
  Complex to Magnitude-Angle : ComplexToMagnitudeAngle  Output=Angle
  "Filter " : Subsystem
  Real-Imag to Complex : RealImagToComplex
  Subtract : Sum  Inputs=+-
  Subtract1 : Sum  Inputs=+-
  Heading : Outport
  wires:
  Pos midden achter 2/1 -> Subtract/2
  "Pos voor 2 "/1 -> Subtract/1
  Pos voor 1/1 -> Subtract1/1
  Pos midden achter 1/1 -> Subtract1/2
  Real-Imag to Complex/1 -> Complex to Magnitude-Angle/1
  Complex to Magnitude-Angle/1 -> "Filter "/1(In1)
  Subtract/1 -> Real-Imag to Complex/1
  Subtract1/1 -> Real-Imag to Complex/2
  "Filter "/1(Out1) -> Heading/1

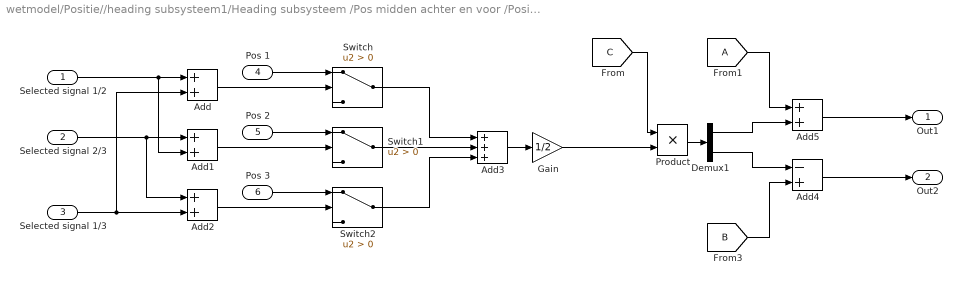
== system wetmodel/Positie//heading subsysteem1/Heading subsysteem /Pos midden achter en voor /Positie midden achter ==
  Selected signal 1/2 : Inport
  Selected signal 2/3 : Inport  Port=2
  Selected signal 1/3 : Inport  Port=3
  "Pos 1 " : Inport  Port=4
  "Pos 2 " : Inport  Port=5
  "Pos 3 " : Inport  Port=6
  Add{,1..2,5} (4 alike) : Sum
  Add3 : Sum  Inputs=+++
  Add4 : Sum  Inputs=-+
  Demux1 : Demux  Outputs=2
  Gain : Gain  Gain=1/2
  Product : Product
  Switch : Switch  Criteria=u2 > Threshold
  Switch1 : Switch  Criteria=u2 > Threshold
  Switch2 : Switch  Criteria=u2 > Threshold
  Out1 : Outport
  Out2 : Outport  Port=2
  wires:
  Add/1 -> Switch/2
  Add1/1 -> Switch1/2
  Add2/1 -> Switch2/2
  Selected signal 1/2/1 -> Add/1, Add1/2
  Selected signal 2/3/1 -> Add1/1, Add2/1
  Selected signal 1/3/1 -> Add/2, Add2/2
  Switch/1 -> Add3/1
  Switch1/1 -> Add3/2
  Switch2/1 -> Add3/3
  Add3/1 -> Gain/1
  Gain/1 -> Product/2
  [C] -> Product/1
  [A] -> Add5/1
  [B] -> Add4/2
  Add5/1 -> Out1/1
  Add4/1 -> Out2/1
  "Pos 1 "/1 -> Switch/1
  "Pos 2 "/1 -> Switch1/1
  "Pos 3 "/1 -> Switch2/1
  Demux1/1 -> Add5/2
  Demux1/2 -> Add4/1
  Product/1 -> Demux1/1

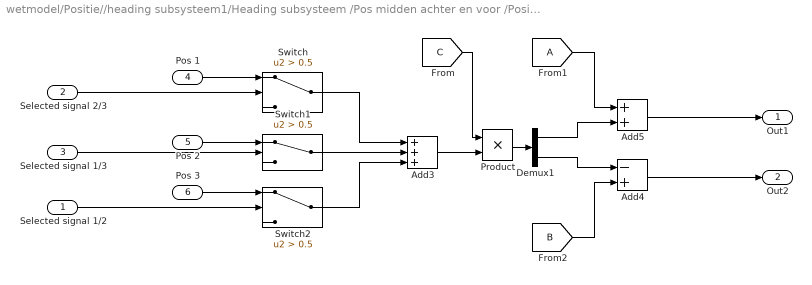
== system wetmodel/Positie//heading subsysteem1/Heading subsysteem /Pos midden achter en voor /Positie voor ==
  Selected signal 1/2 : Inport
  Selected signal 2/3 : Inport  Port=2
  Selected signal 1/3 : Inport  Port=3
  "Pos 1 " : Inport  Port=4
  "Pos 2 " : Inport  Port=5
  "Pos 3 " : Inport  Port=6
  Add3 : Sum  Inputs=+++
  Add4 : Sum  Inputs=-+
  Add5 : Sum
  Demux1 : Demux  Outputs=2
  Product : Product
  Switch : Switch  Criteria=u2 > Threshold  Threshold=0.5
  Switch1 : Switch  Criteria=u2 > Threshold  Threshold=0.5
  Switch2 : Switch  Criteria=u2 > Threshold  Threshold=0.5
  Out1 : Outport
  Out2 : Outport  Port=2
  wires:
  Switch/1 -> Add3/1
  Switch1/1 -> Add3/2
  Switch2/1 -> Add3/3
  [C] -> Product/1
  [A] -> Add5/1
  [B] -> Add4/2
  Add5/1 -> Out1/1
  Add4/1 -> Out2/1
  Selected signal 2/3/1 -> Switch/2
  Selected signal 1/2/1 -> Switch2/2
  Selected signal 1/3/1 -> Switch1/2
  "Pos 1 "/1 -> Switch/1
  "Pos 2 "/1 -> Switch1/1
  "Pos 3 "/1 -> Switch2/1
  Product/1 -> Demux1/1
  Demux1/1 -> Add5/2
  Demux1/2 -> Add4/1
  Add3/1 -> Product/2

== system wetmodel/Positie//heading subsysteem1/Heading subsysteem /heading/Filter  ==
  In1 : Inport
  Constant2 : Constant  Value=3
  Relational Operator2 : RelationalOperator  Operator===  OutDataTypeStr=boolean  RndMeth=Nearest
  Sample and Hold1 : powerlib_meascontrol/Additional Components/Sample and Hold  ic=0  Ts=0
      settings: SourceProductName=Simscape Electrical  SourceProductBaseCode=PS
  Out1 : Outport
  wires:
  In1/1 -> Sample and Hold1/1
  Sample and Hold1/1 -> Out1/1
  [E] -> Relational Operator2/1
  Relational Operator2/1 -> Sample and Hold1/2
  Constant2/1 -> Relational Operator2/2
